simulink library "Lib_DQTrans_dqe2dqs"  (R2021a)
settings: Solver=VariableStepAuto  StartTime=0.0  StopTime=10.0  RelTol=1e-3
settings Model: Creator=30610  LastModifiedBy=30610

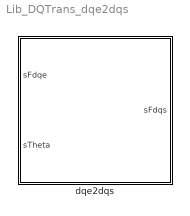
== system Lib_DQTrans_dqe2dqs ==
  dqe2dqs : Subsystem

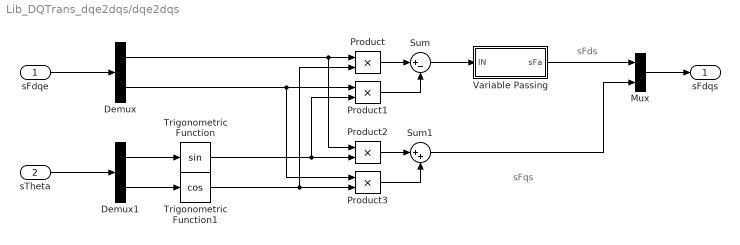
== system Lib_DQTrans_dqe2dqs/dqe2dqs ==
  note: sFds
  note: sFqs
  sFdqe : Inport
  sTheta : Inport  Port=2
  Demux : Demux  Outputs=2
  Demux1 : Demux  Outputs=2
  Mux : Mux  Inputs=2
  Product{,1..3} (4 alike) : Product  RndMeth=Zero
  Sum : Sum  Inputs=|+-
  Sum1 : Sum  Inputs=|++
  Trigonometric Function : Trigonometry
  Trigonometric Function1 : Trigonometry  Operator=cos
  Variable Passing : Stateflow chart  TreatAsAtomicUnit=on
  sFdqs : Outport  VectorParamsAs1DForOutWhenUnconnected=off
  wires:
  Mux/1 -> sFdqs/1
  sTheta/1 -> Demux1/1
  Demux/1 -> Product2/1, Product/1
  Demux/2 -> Product3/1, Product1/1
  Sum/1 -> Variable Passing/1(IN)
  Demux1/1 -> Trigonometric Function/1
  Product2/1 -> Sum1/1
  Demux1/2 -> Trigonometric Function1/1
  Sum1/1 -> Mux/2
  Product1/1 -> Sum/2
  Product3/1 -> Sum1/2
  sFdqe/1 -> Demux/1
  Product/1 -> Sum/1
  Variable Passing/1(sFa) -> Mux/1
  Trigonometric Function/1 -> Product1/2, Product2/2
  Trigonometric Function1/1 -> Product/2, Product3/2

== stateflow chart Lib_DQTrans_dqe2dqs/dqe2dqs/Variable Passing ==
  (default) -> (junction 3)
  (junction 3) -> (junction 5) : {sFa = IN;}
  (junction 5) -> (junction 6)
  data: IN input; sFa output single
